simulink model "RCAm_model_run"  (R2026a)
settings: Solver=VariableStepAuto  StopTime=180
values from neighbouring files (symbols this model uses):
  x0 = [85 ... (first row only)    [initialize_constants.m]
undefined symbols (not defined in the file or in its folder): RCAM_model
settings Model: NumberOfSteps=5  Creator=Admin  LastModifiedBy=Admin

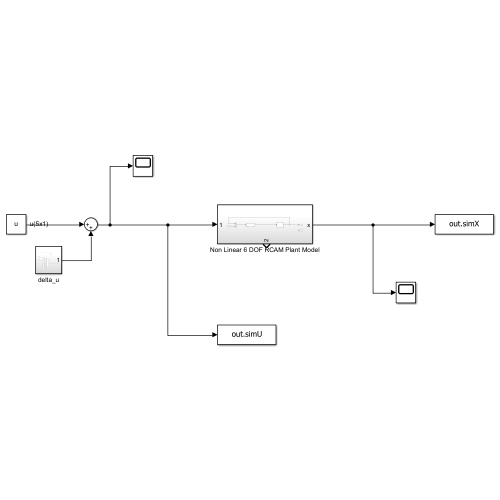
[thumbnail: Simulink's stored preview of the top-level diagram]
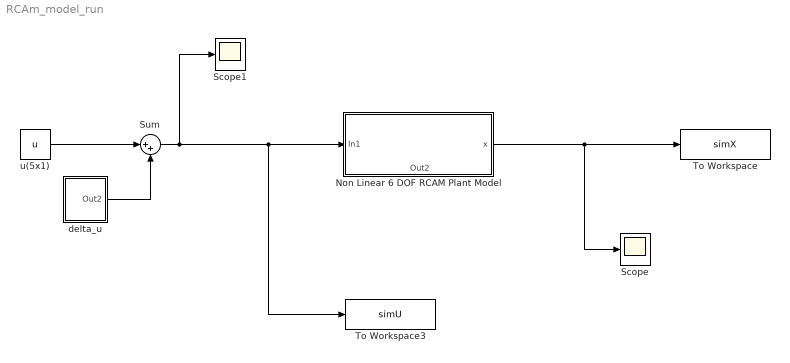
== system RCAm_model_run ==
  Non Linear 6 DOF RCAM Plant Model : Subsystem
      settings: PortSchema="{\"entries\":[{\"content\":{\"sides\":[{\"content\":{\"connectorIds\":[\"In1\"]},\"type\":\"ConnectorPlacement.EquallySpacedRectSide\",\"uuid\":\"caba342f-2d80-4c10-98a3-49ebc2ccef59\"},{\"content\":{\"connectorIds\":[\"Out1\"],\"side\":\"RIGHT\"},\"type\":\"ConnectorPlacement.EquallySpacedRectSide\",\"uuid\":\"3e3511b8-a300-467a-bfc2-d64d2a475386\"},{\"content\":{\"side\":\"TOP\"},\"type\":\"ConnectorPlacement.EquallySpacedRectSide\",\"uuid\":\"73f36e6a-95e5-4827-a6ce-df9d27ce76c1\"},{\"content\":{\"connectorIds\":[\"Out2\"],\"side\":\"BOTTOM\"},\"type\":\"ConnectorPlacement.EquallySpacedRectSide\",\"uuid\":\"e55f739f-c353-4d87-9f02-967734aee642\"}]},\"type\":\"ConnectorPlacement.EquallySpacedConnector\",\"uuid\":\"fbb9a17d-b0c3-4e53-99d0-10adc0e5ed33\"}],\"packageUris\":[\"http://schema.mathworks.com/mf0/Connector/R2020b\"],\"version\":\"1.0\"}"
  Scope : Scope
  Scope1 : Scope
  Sum : Sum  Inputs=|++
  To Workspace : ToWorkspace  VariableName=simX  SaveFormat=Timeseries  SampleTime=-1
  To Workspace3 : ToWorkspace  VariableName=simU  SaveFormat=Timeseries  SampleTime=-1
  delta_u : Subsystem
  u(5x1) : Constant  Value=u
  wires:
  Non Linear 6 DOF RCAM Plant Model/1(x) -> Scope/1, To Workspace/1
  u(5x1)/1 -> Sum/1
  delta_u/1(Out2) -> Sum/2
  Sum/1 -> Scope1/1, To Workspace3/1, Non Linear 6 DOF RCAM Plant Model/1(In1)

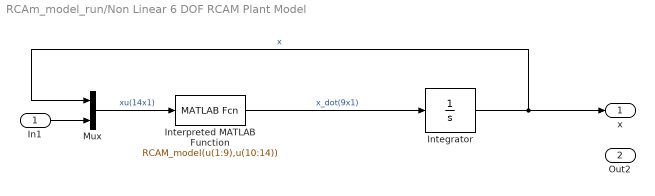
== system RCAm_model_run/Non Linear 6 DOF RCAM Plant Model ==
  In1 : Inport
  Integrator : Integrator  InitialCondition=x0
  Interpreted MATLAB Function : MATLABFcn  MATLABFcn=RCAM_model(u(1:9),u(10:14))
  Mux : Mux  Inputs=2
  x : Outport
  Out2 : Outport  Port=2
  wires:
  Interpreted MATLAB Function/1 -> Integrator/1  "x_dot(9x1)"
  Integrator/1 -> x/1, Mux/1  "x"
  In1/1 -> Mux/2
  Mux/1 -> Interpreted MATLAB Function/1  "xu(14x1)"

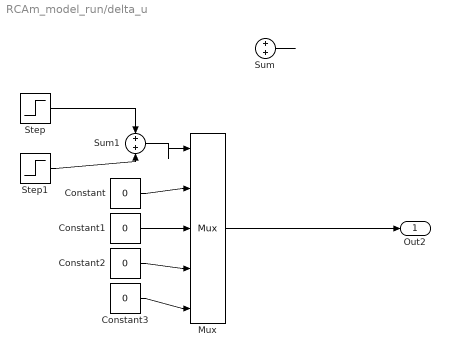
== system RCAm_model_run/delta_u ==
  Constant{,1..3} (4 alike) : Constant  Value=0
  Mux : Mux  Inputs=5
  Step : Step  Time=30  FinalValue=5*pi/180  SampleTime=0
  Step1 : Step  Time=30+2  FinalValue=-5*pi/180  SampleTime=0
  Sum : Sum
  Sum1 : Sum
  Out2 : Outport
  wires:
  ? -> Sum/1
  Sum1/1 -> Mux/1
  ? -> Sum/2
  Step/1 -> Sum1/1
  Constant1/1 -> Mux/3
  Constant2/1 -> Mux/4
  Constant/1 -> Mux/2
  Step1/1 -> Sum1/2
  Constant3/1 -> Mux/5
  Sum/1 -> ?
  Mux/1 -> Out2/1
